simulink library "LumAerospaceBlockset_EquationsOfMotion"  (R2021a)
settings: Solver=ode45  StartTime=0.0  StopTime=10.0  RelTol=1e-3  EnableMultiTasking=on
values from neighbouring files (symbols this model uses):
  Xgeodetic0 = [lat0;lon0;h0]    [MAIN_RCAMDemo.m]
libraries: LumAerospaceBlockset_Utilities x3
settings Model: Creator=Christopher  LastModifiedBy=chris
settings SolverCC: AlgebraicLoopSolver=TrustRegion
settings DataIOCC: LimitDataPoints=on  SaveFormat=Array  ReturnWorkspaceOutputs=off
settings OptimizationCC: LifeSpan=inf
settings DebuggingCC: SolverPrmCheckMsg=warning  SFUnexpectedBacktrackingDiag=warning  SFNoUnconditionalDefaultTransitionDiag=warning  SFExecutionAtInitializationDiag=none  SFMachineParentedDataDiag=warning  ArithmeticOperatorsInVariantConditions=warning
settings HardwareCC: ProdBitPerPointer=32  ProdBitPerSizeT=32  ProdBitPerPtrDiffT=32  ProdLargestAtomicFloat=None  ProdIntDivRoundTo=Undefined  ProdEndianess=Unspecified  ProdWordSize=32  ProdHWDeviceType=32-bit Generic
settings ModelReferenceCC: PropagateSignalLabelsOutOfModel=off
settings SFSimCC: SimUseLocalCustomCode=off  CustomCodeUndefinedFunction=UseInterfaceOnly
settings RTWCC: RTWUseLocalCustomCode=off
settings CodeAppCC: StateflowObjectComments=on
settings GRTTargetCC: TargetLangStandard=C89/C90 (ANSI)
settings ConfigComp: CovMetricSettings=dw  CovSaveCumulativeToWorkspaceVar=on  CovSaveSingleToWorkspaceVar=on  CovExternalEMLEnable=off  CovSFcnEnable=off

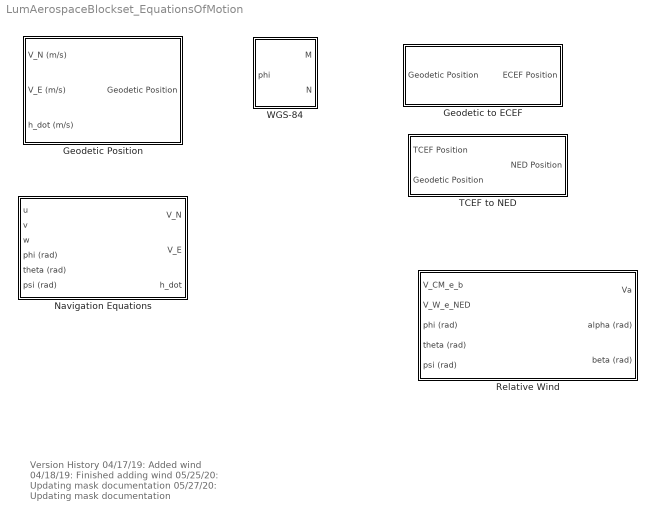
== system LumAerospaceBlockset_EquationsOfMotion ==
  note: Version History
      | 04/17/19: Added wind
      | 04/18/19: Finished adding wind
      | 05/25/20: Updating mask documentation
      | 05/27/20: Updating mask documentation
  Geodetic Position : Subsystem  mask{Xgeodetic0=Xgeodetic0}
      mask prompts: Xgeodetic0 "Initial Position (Geodetic)"
      mask help:
      | Obtains the position in Geodetic Coordinates from North-East-Down velocities.
      |
      | Longitude is bounded between [-pi,pi).  Latitutde is unbounded.  This creates problems near phi=+/-pi/2.  This block should not be used near these limits (ie north/south pole)
      |
      | Inputs are velocities in North-East-Down frame (except for h_dot = -V_down).    All inputs must be in units of meters/sec.
      |
      | Inputs:	V_N:	North velocity (m/s)
      | 	V_E:	East velocity (m/s)
      | 	h_dot:	Altitude_dot (m/s)
      |
      | Outputs:	3x1 vector of (phi;lambda;h).
      | 		phi = geodetic latitude (rad)
      | 		lambda = terrestrial longitude (rad)
      | 		h = geodetic altitude (m)
      |
      | For more information, see Stevens, B.L., Lewis, F.L., "Aircraft Control and Simulation 2nd Ed".  2003 John Wiley & Sons.  Pg. 37
      |
      | Christopher Lum
      | lum@uw.edu
  Geodetic to ECEF : Subsystem  Description=|
      | Version History  
      |                  
      | 05/??/05: Created
      mask help:
      | Convert from geodetic coordinates to Earth-Centered-Earth-Fixed (ECEF) frame.
      |
      | Inputs:		Geodetic Position:	3x1 vector of [phi;lambda;h].
      |
      | Outputs:	ECEF position:		3x1 vector of [x_ECEF;y_ECEF;z_ECEF].
      |
      | For more information, see Stevens, B.L., Lewis, F.L., "Aircraft Control and Simulation 2nd Ed".  2003 John Wiley & Sons.  Pg. 38
      |
      | Created by Christopher Lum
      | lum@u.washington.edu
  Navigation Equations : Subsystem  Description=|
      | Version History  
      |                  
      | 05/24/05: Created
      mask help:
      | Converts velocities in body frame to velocities in North-East-Down frame.  This computes the outputs using the following equations
      |
      | 	V_N = u*cos(theta)*cos(psi)+v*(-cos(phi)*sin(psi)+sin(phi)*sin(theta)*cos(psi))+w*(sin(phi)*sin(psi)+cos(phi)*sin(theta)*cos(psi))
      |
      | 	V_E = u*cos(theta)*sin(psi)+v*(cos(phi)*cos(psi)+sin(phi)*sin(theta)*sin(psi))+w*(-sin(phi)*cos(psi)+cos(phi)*sin(theta)*sin(psi))
      |
      | 	h_dot = u*sin(theta)-v*sin(phi)*cos(theta)-w*cos(phi)*cos(theta)
      |
      | Note that h_dot = -V_down
      |
      | Inputs:		u:	body velocity x
      | 		v:	body velocity y
      | 		w:	body velocity z
      | 		phi:	Euler angle bank (rad)
      | 		theta:	Euler angle pitch (rad)
      | 		psi:	Euler angle yaw (rad)
      |
      | Outputs:		V_N:	velocity north
      | 		V_E:	velocity east
      | 		h_dot:	altitude rate of change (positive h_dot implies climb)
      |
      | For more information, see Stevens, B.L., Lewis, F.L., "Aircraft Control and Simulation 2nd Ed". 2003 John Wiley & Sons. Pg.110
      |
      | Christopher Lum
      | lum@uw.edu
  Relative Wind : Subsystem
      mask help:
      | Computes the airspeed, angle of attack, and angle of sideslip experienced by an aircraft in a steady wind field.
      |
      | 	v_CM_e_b = [u;v;w]
      | 	V_W_e_NED   = [W_N; W_E; W_D]
      |
      | For example, if the wind is directly from the South (in other words it is blowing directly North) and 10 m/s, then V_W_e_n = [10; 0; 0].
      |
      | If there is no relative motion (V_CM_e_b = V_W_e_NED) then alpha and beta are set to 0 (as opposed to NaN).
      |
      | Inputs:	V_CM_e_b:	velocity vector of CM of aircraft w.r.t. earth/inertial frame expressed in the body (b) frame (3x1 vector)
      | 	V_W_e_NED:	velocity vector of the wind w.r.t. earth/inertial frame expressed in the north, east, down (NED) frame (3x1)
      | 	phi:	Euler angle bank (rad)
      | 	theta:	Euler angle pitch (rad)
      | 	psi:	Euler angle yaw (rad)
      |
      | Outputs:	Va:	airspeed experienced by the aircraft
      | 	alpha:	angle of attack experienced by aircraft (rad)
      | 	beta:	angle of sideslip experienced by aircraft (rad)
      |
      | Created by Christopher Lum
      | lum@uw.edu
      mask Display: image('WindIcon.png')
  TCEF to NED : Subsystem  Description=|
      | Version History  
      |                  
      | 05/??/05: Created
      mask help:
      | Convert from Target-Centered-Earth-Fixed (TCEF) frame to North-East-Down (NED) frame.  TCEF frame is same as ECEF frame except its origin is at target specified by phi, lambda, and h.
      |
      | Inputs:		TCEF Position:		3x1 vector of [x_TCEF;y_TCEF;z_TCEF].
      | 		Geodetic Position:	3x1 vector of [phi;lambda;h].
      |
      | Outputs:	NED position:		3x1 vector of [PN,PE,PD]
      |
      | For more information, see Stevens, B.L., Lewis, F.L., "Aircraft Control and Simulation 2nd Ed".  2003 John Wiley & Sons.  Pg. 37
      |
      | Created by Christopher Lum
      | lum@u.washington.edu
  WGS-84 : Subsystem  Description=|
      | Version History  
      |                  
      | 05/??/05: Created
      mask help:
      | Calculates the meridian raidus of curvature (M), and the prime vertical radius of curvature (N).
      |
      | Inputs:	phi:	Geodetic latitude (rad)
      |
      | Outputs:	M:	Meridian radius of curvature (m)
      | 	N:	Prime vertical radius of curvature (m)
      |
      | For more information, see Stevens, B.L., Lewis, F.L., "Aircraft Control and Simulation 2nd Ed".  2003 John Wiley & Sons.  Pg. 37
      |
      | Christopher Lum
      | lum@uw.edu

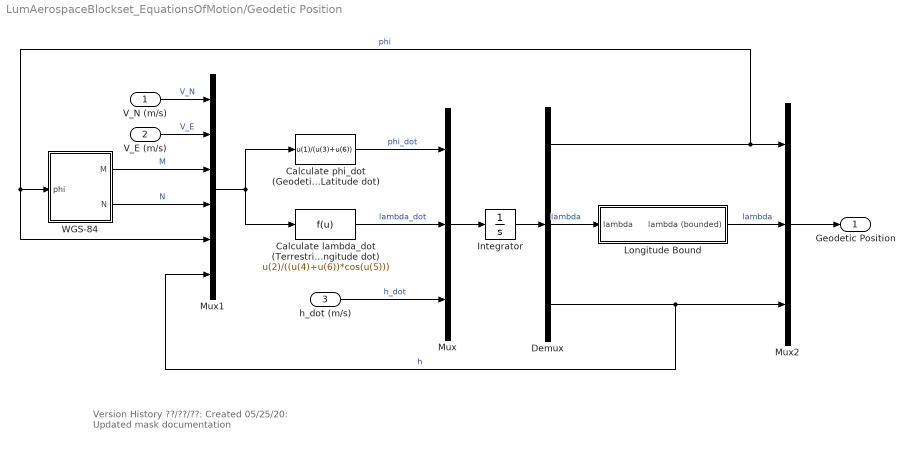
== system LumAerospaceBlockset_EquationsOfMotion/Geodetic Position ==
  note: Version History
      | ??/??/??: Created
      | 05/25/20: Updated mask documentation
  V_N (m/s) : Inport
  V_E (m/s) : Inport  Port=2
  h_dot (m/s) : Inport  Port=3
  Calculate lambda_dot (Terrestrial Longitude dot) : Fcn  Expr=u(2)/((u(4)+u(6))*cos(u(5)))
  Calculate phi_dot (Geodetic Latitude dot) : Fcn  Expr=u(1)/(u(3)+u(6))
  Demux : Demux  Outputs=3
  Integrator : Integrator  InitialCondition=Xgeodetic0
  Longitude Bound : Subsystem
      mask help:
      | Converts input longitude to it equivalent in the range [-pi,pi).
      |
      | Original Block concept from Aerosim Blockset by Unmanned Dynamics.  www.u-dynamics.com
  Mux : Mux  Inputs=3
  Mux1 : Mux  Inputs=6
  Mux2 : Mux  Inputs=3
  WGS-84 : Subsystem
  Geodetic Position : Outport  VectorParamsAs1DForOutWhenUnconnected=off
  wires:
  Longitude Bound/1(lambda (bounded)) -> Mux2/2  "lambda"
  Mux1/1 -> Calculate lambda_dot (Terrestrial Longitude dot)/1, Calculate phi_dot (Geodetic Latitude dot)/1
  Calculate phi_dot (Geodetic Latitude dot)/1 -> Mux/1  "phi_dot"
  Calculate lambda_dot (Terrestrial Longitude dot)/1 -> Mux/2  "lambda_dot"
  WGS-84/2(N) -> Mux1/4  "N"
  WGS-84/1("M ") -> Mux1/3  "M"
  h_dot (m/s)/1 -> Mux/3  "h_dot"
  V_E (m/s)/1 -> Mux1/2  "V_E"
  V_N (m/s)/1 -> Mux1/1  "V_N"
  Demux/3 -> Mux1/6, Mux2/3  "h"
  Demux/2 -> Longitude Bound/1(lambda)  "lambda"
  Demux/1 -> Mux1/5, WGS-84/1(phi), Mux2/1  "phi"
  Integrator/1 -> Demux/1
  Mux/1 -> Integrator/1
  Mux2/1 -> Geodetic Position/1

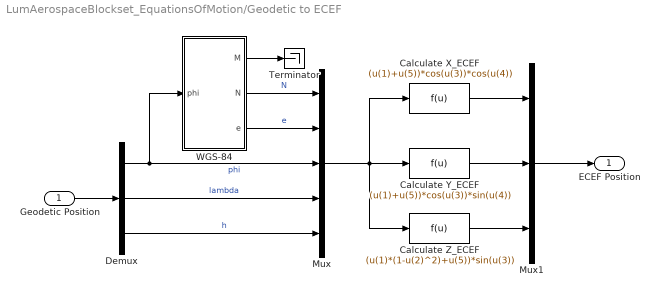
== system LumAerospaceBlockset_EquationsOfMotion/Geodetic to ECEF ==
  Geodetic Position : Inport
  Calculate X_ECEF : Fcn  Expr=(u(1)+u(5))*cos(u(3))*cos(u(4))
  Calculate Y_ECEF : Fcn  Expr=(u(1)+u(5))*cos(u(3))*sin(u(4))
  Calculate Z_ECEF : Fcn  Expr=(u(1)*(1-u(2)^2)+u(5))*sin(u(3))
  Demux : Demux  Outputs=3
  Mux : Mux  Inputs=5
  Mux1 : Mux  Inputs=3
  Terminator : Terminator
  WGS-84 : Subsystem
  ECEF Position : Outport  VectorParamsAs1DForOutWhenUnconnected=off
  wires:
  Geodetic Position/1 -> Demux/1
  Mux/1 -> Calculate Y_ECEF/1, Calculate X_ECEF/1, Calculate Z_ECEF/1
  Calculate X_ECEF/1 -> Mux1/1
  Calculate Y_ECEF/1 -> Mux1/2
  Calculate Z_ECEF/1 -> Mux1/3
  Mux1/1 -> ECEF Position/1
  Demux/2 -> Mux/4  "lambda"
  Demux/3 -> Mux/5  "h"
  WGS-84/2(N) -> Mux/1  "N"
  WGS-84/3(e) -> Mux/2  "e"
  Demux/1 -> Mux/3, WGS-84/1(phi)  "phi"
  WGS-84/1("M ") -> Terminator/1

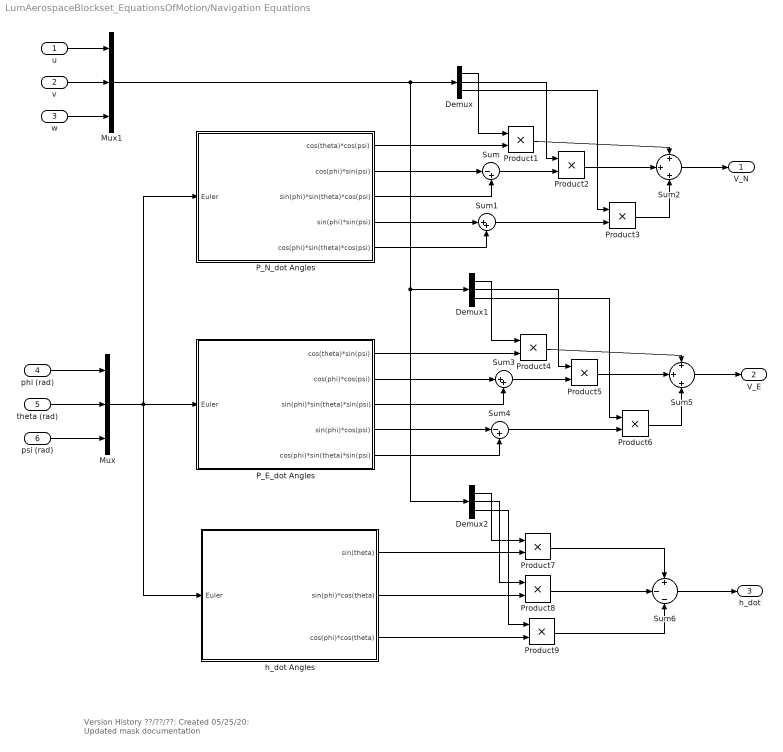
== system LumAerospaceBlockset_EquationsOfMotion/Navigation Equations ==
  note: Version History
      | ??/??/??: Created
      | 05/25/20: Updated mask documentation
  u : Inport
  v : Inport  Port=2
  w : Inport  Port=3
  phi (rad) : Inport  Port=4
  theta (rad) : Inport  Port=5
  psi (rad) : Inport  Port=6
  Demux : Demux  Outputs=3
  Demux1 : Demux  Outputs=3
  Demux2 : Demux  Outputs=3
  Mux : Mux  Inputs=3
  Mux1 : Mux  Inputs=3
  P_E_dot Angles : Subsystem
  P_N_dot Angles : Subsystem
  Product{1..9} (9 alike) : Product  RndMeth=Zero
  Sum : Sum  Inputs=|-+
  Sum1 : Sum  Inputs=|++
  Sum2 : Sum  Inputs=+|+|+
  Sum3 : Sum  Inputs=|++
  Sum4 : Sum  Inputs=|-+
  Sum5 : Sum  Inputs=+|+|+
  Sum6 : Sum  Inputs=+|-|-
  h_dot Angles : Subsystem
  V_N : Outport  VectorParamsAs1DForOutWhenUnconnected=off
  V_E : Outport  Port=2  VectorParamsAs1DForOutWhenUnconnected=off
  h_dot : Outport  Port=3  VectorParamsAs1DForOutWhenUnconnected=off
  wires:
  Sum6/1 -> h_dot/1
  Product9/1 -> Sum6/3
  Product8/1 -> Sum6/2
  Product7/1 -> Sum6/1
  h_dot Angles/3(cos(phi)*cos(theta)) -> Product9/2
  Demux2/3 -> Product9/1
  h_dot Angles/2(sin(phi)*cos(theta)) -> Product8/2
  Demux2/2 -> Product8/1
  h_dot Angles/1(sin(theta)) -> Product7/2
  Demux2/1 -> Product7/1
  P_E_dot Angles/5(cos(phi)*sin(theta)*sin(psi)) -> Sum4/2
  P_E_dot Angles/4(sin(phi)*cos(psi)) -> Sum4/1
  P_E_dot Angles/3(sin(phi)*sin(theta)*sin(psi)) -> Sum3/2
  P_E_dot Angles/2(cos(phi)*cos(psi)) -> Sum3/1
  P_E_dot Angles/1(cos(theta)*sin(psi)) -> Product4/2
  Demux1/3 -> Product6/1
  Demux1/2 -> Product5/1
  Demux1/1 -> Product4/1
  Sum5/1 -> V_E/1
  Product6/1 -> Sum5/3
  Product5/1 -> Sum5/2
  Product4/1 -> Sum5/1
  Sum4/1 -> Product6/2
  Sum3/1 -> Product5/2
  Demux/3 -> Product3/1
  Demux/2 -> Product2/1
  Demux/1 -> Product1/1
  Mux1/1 -> Demux2/1, Demux1/1, Demux/1
  w/1 -> Mux1/3
  v/1 -> Mux1/2
  u/1 -> Mux1/1
  Sum2/1 -> V_N/1
  Product3/1 -> Sum2/3
  Product2/1 -> Sum2/2
  Product1/1 -> Sum2/1
  Sum1/1 -> Product3/2
  P_N_dot Angles/5(cos(phi)*sin(theta)*cos(psi)) -> Sum1/2
  P_N_dot Angles/4(sin(phi)*sin(psi)) -> Sum1/1
  Sum/1 -> Product2/2
  P_N_dot Angles/3(sin(phi)*sin(theta)*cos(psi)) -> Sum/2
  P_N_dot Angles/2("cos(phi)*sin(psi) ") -> Sum/1
  P_N_dot Angles/1(cos(theta)*cos(psi)) -> Product1/2
  Mux/1 -> h_dot Angles/1(Euler), P_E_dot Angles/1(Euler), P_N_dot Angles/1(Euler)
  psi (rad)/1 -> Mux/3
  theta (rad)/1 -> Mux/2
  phi (rad)/1 -> Mux/1

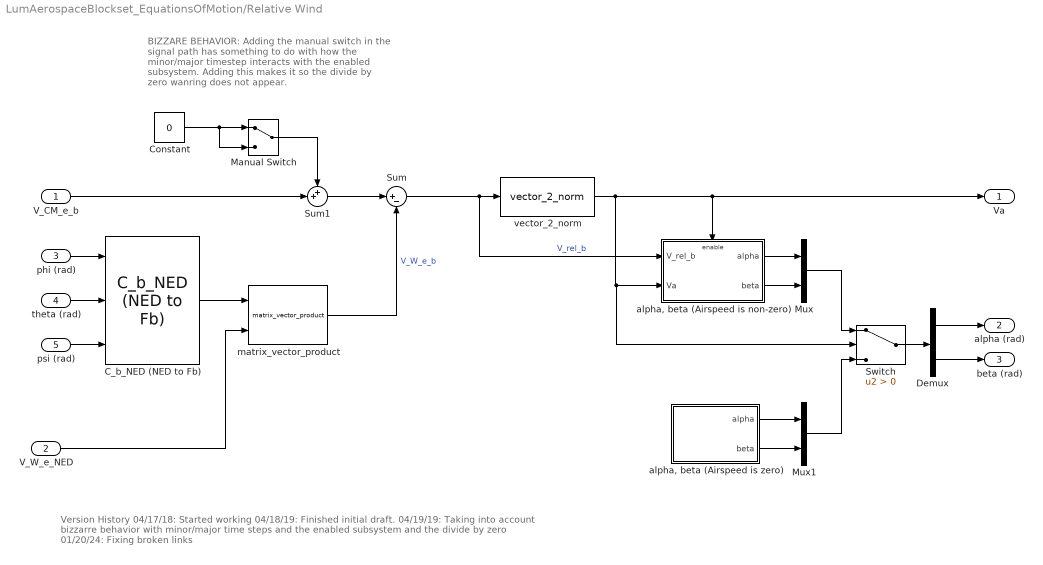
== system LumAerospaceBlockset_EquationsOfMotion/Relative Wind ==
  note: BIZZARE BEHAVIOR: Adding the manual switch in the signal path has something to do with how the minor/major timestep interacts with the enabled subsystem. Adding this makes it so the divide by zero wanring does not appear.
  note: Version History
      | 04/17/18: Started working
      | 04/18/19: Finished initial draft.
      | 04/19/19: Taking into account bizzarre behavior with minor/major time steps and the enabled subsystem and the divide by zero
      | 01/20/24: Fixing broken links
  V_CM_e_b : Inport
  V_W_e_NED : Inport  Port=2
  phi (rad) : Inport  Port=3
  theta (rad) : Inport  Port=4
  psi (rad) : Inport  Port=5
  C_b_NED (NED to Fb) : LumAerospaceBlockset_Utilities/C_b_NED (NED to Fb)
  Constant : Constant  Value=0
  Demux : Demux  Outputs=2
  Manual Switch : ManualSwitch
  Mux : Mux  Inputs=2
  Mux1 : Mux  Inputs=2
  Sum : Sum  Inputs=|+-
  Sum1 : Sum  Inputs=++|
  Switch : Switch  Criteria=u2 > Threshold
  "alpha, beta (Airspeed is non-zero)" : Subsystem
  "alpha, beta (Airspeed is zero)" : Subsystem
  matrix_vector_product : LumAerospaceBlockset_Utilities/matrix_vector_product
  vector_2_norm : LumAerospaceBlockset_Utilities/vector_2_norm
  Va : Outport  VectorParamsAs1DForOutWhenUnconnected=off
  alpha (rad) : Outport  Port=2  VectorParamsAs1DForOutWhenUnconnected=off
  beta (rad) : Outport  Port=3  VectorParamsAs1DForOutWhenUnconnected=off
  wires:
  V_W_e_NED/1 -> matrix_vector_product/2
  V_CM_e_b/1 -> Sum1/2
  Sum/1 -> "alpha, beta (Airspeed is non-zero)"/1(V_rel_b), vector_2_norm/1  "V_rel_b"
  psi (rad)/1 -> C_b_NED (NED to Fb)/3
  phi (rad)/1 -> C_b_NED (NED to Fb)/1
  theta (rad)/1 -> C_b_NED (NED to Fb)/2
  C_b_NED (NED to Fb)/1 -> matrix_vector_product/1
  matrix_vector_product/1 -> Sum/2  "V_W_e_b"
  "alpha, beta (Airspeed is non-zero)"/1(alpha) -> Mux/1
  "alpha, beta (Airspeed is non-zero)"/2(beta) -> Mux/2
  "alpha, beta (Airspeed is zero)"/1(alpha) -> Mux1/1
  "alpha, beta (Airspeed is zero)"/2(beta) -> Mux1/2
  vector_2_norm/1 -> Switch/2, "alpha, beta (Airspeed is non-zero)"/2(Va), Va/1, "alpha, beta (Airspeed is non-zero)"/Enable
  Mux/1 -> Switch/1
  Mux1/1 -> Switch/3
  Switch/1 -> Demux/1
  Demux/1 -> alpha (rad)/1
  Demux/2 -> beta (rad)/1
  Manual Switch/1 -> Sum1/1
  Constant/1 -> Manual Switch/2, Manual Switch/1
  Sum1/1 -> Sum/1

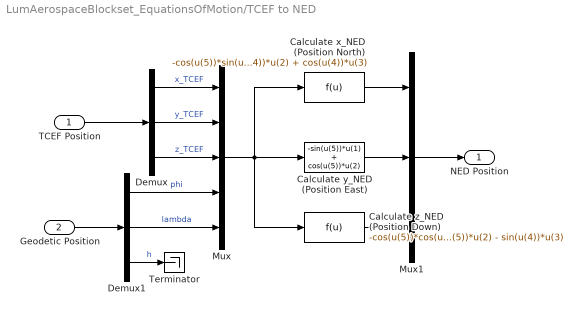
== system LumAerospaceBlockset_EquationsOfMotion/TCEF to NED ==
  TCEF Position : Inport
  Geodetic Position : Inport  Port=2
  Calculate x_NED (Position North) : Fcn  Expr=-cos(u(5))*sin(u(4))*u(1) - sin(u(5))*sin(u(4))*u(2) + cos(u(4))*u(3)
  Calculate y_NED (Position East) : Fcn  Expr=-sin(u(5))*u(1) + cos(u(5))*u(2)
  Calculate z_NED (Position Down) : Fcn  Expr=-cos(u(5))*cos(u(4))*u(1) - cos(u(4))*sin(u(5))*u(2) - sin(u(4))*u(3)
  Demux : Demux  Outputs=3
  Demux1 : Demux  Outputs=3
  Mux : Mux  Inputs=5
  Mux1 : Mux  Inputs=3
  Terminator : Terminator
  NED Position : Outport  VectorParamsAs1DForOutWhenUnconnected=off
  wires:
  TCEF Position/1 -> Demux/1
  Geodetic Position/1 -> Demux1/1
  Demux/1 -> Mux/1  "x_TCEF"
  Demux/2 -> Mux/2  "y_TCEF"
  Demux/3 -> Mux/3  "z_TCEF"
  Demux1/1 -> Mux/4  "phi"
  Demux1/2 -> Mux/5  "lambda"
  Demux1/3 -> Terminator/1  "h"
  Calculate x_NED (Position North)/1 -> Mux1/1
  Calculate y_NED (Position East)/1 -> Mux1/2
  Calculate z_NED (Position Down)/1 -> Mux1/3
  Mux1/1 -> NED Position/1
  Mux/1 -> Calculate y_NED (Position East)/1, Calculate x_NED (Position North)/1, Calculate z_NED (Position Down)/1

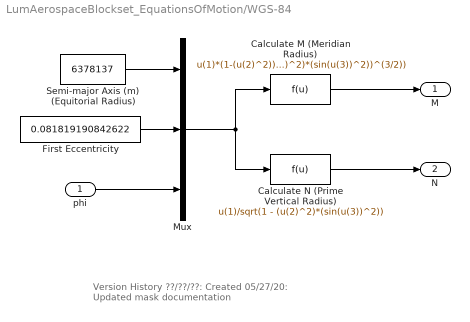
== system LumAerospaceBlockset_EquationsOfMotion/WGS-84 ==
  note: Version History
      | ??/??/??: Created
      | 05/27/20: Updated mask documentation
  phi : Inport
  Calculate M (Meridian Radius) : Fcn  Expr=u(1)*(1-(u(2)^2))/((1-(u(2)^2)*(sin(u(3))^2))^(3/2))
  Calculate N (Prime Vertical Radius) : Fcn  Expr=u(1)/sqrt(1 - (u(2)^2)*(sin(u(3))^2))
  First Eccentricity : Constant  Value=0.081819190842622
  Mux : Mux  Inputs=3
  "Semi-major Axis (m) (Equitorial Radius) " : Constant  Value=6378137
  "M " : Outport  VectorParamsAs1DForOutWhenUnconnected=off
  N : Outport  Port=2  VectorParamsAs1DForOutWhenUnconnected=off
  wires:
  "Semi-major Axis (m) (Equitorial Radius) "/1 -> Mux/1
  First Eccentricity/1 -> Mux/2
  Calculate M (Meridian Radius)/1 -> "M "/1
  phi/1 -> Mux/3
  Calculate N (Prime Vertical Radius)/1 -> N/1
  Mux/1 -> Calculate N (Prime Vertical Radius)/1, Calculate M (Meridian Radius)/1

== system LumAerospaceBlockset_EquationsOfMotion/Geodetic Position/Longitude Bound ==
  lambda : Inport
  2pi : Constant  Value=2*pi
  Math Function : Math  Operator=mod  SignedPower=on  SaturateOnIntegerOverflow=on
  Sum1 : Sum  Inputs=|+-  InputSameDT=on  SaturateOnIntegerOverflow=on  OutDataTypeStr=Inherit: Same as first input
  Sum2 : Sum  Inputs=|++  InputSameDT=on  SaturateOnIntegerOverflow=on  OutDataTypeStr=Inherit: Same as first input
  pi : Constant  Value=pi
  lambda (bounded) : Outport  VectorParamsAs1DForOutWhenUnconnected=off
  wires:
  Sum1/1 -> lambda (bounded)/1
  lambda/1 -> Sum2/1
  pi/1 -> Sum1/2, Sum2/2
  Sum2/1 -> Math Function/1
  2pi/1 -> Math Function/2
  Math Function/1 -> Sum1/1

== system LumAerospaceBlockset_EquationsOfMotion/Geodetic Position/WGS-84 ==
  phi : Inport
  Calculate M (Meridian Radius) : Fcn  Expr=u(1)*(1-(u(2)^2))/((1-(u(2)^2)*(sin(u(3))^2))^(3/2))
  Calculate N (Prime Vertical Radius) : Fcn  Expr=u(1)/sqrt(1 - (u(2)^2)*(sin(u(3))^2))
  First Eccentricity : Constant  Value=0.081819190842622
  Mux : Mux  Inputs=3
  "Semi-major Axis (m) (Equitorial Radius) " : Constant  Value=6378137
  "M " : Outport  VectorParamsAs1DForOutWhenUnconnected=off
  N : Outport  Port=2  VectorParamsAs1DForOutWhenUnconnected=off
  wires:
  Mux/1 -> Calculate M (Meridian Radius)/1, Calculate N (Prime Vertical Radius)/1
  Calculate N (Prime Vertical Radius)/1 -> N/1
  phi/1 -> Mux/3
  Calculate M (Meridian Radius)/1 -> "M "/1
  First Eccentricity/1 -> Mux/2
  "Semi-major Axis (m) (Equitorial Radius) "/1 -> Mux/1

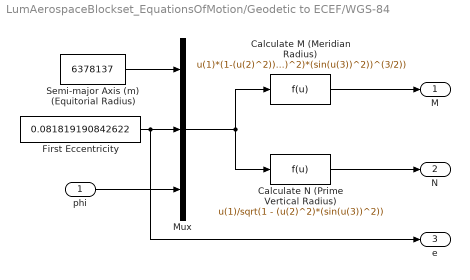
== system LumAerospaceBlockset_EquationsOfMotion/Geodetic to ECEF/WGS-84 ==
  phi : Inport
  Calculate M (Meridian Radius) : Fcn  Expr=u(1)*(1-(u(2)^2))/((1-(u(2)^2)*(sin(u(3))^2))^(3/2))
  Calculate N (Prime Vertical Radius) : Fcn  Expr=u(1)/sqrt(1 - (u(2)^2)*(sin(u(3))^2))
  First Eccentricity : Constant  Value=0.081819190842622
  Mux : Mux  Inputs=3
  "Semi-major Axis (m) (Equitorial Radius) " : Constant  Value=6378137
  "M " : Outport  VectorParamsAs1DForOutWhenUnconnected=off
  N : Outport  Port=2  VectorParamsAs1DForOutWhenUnconnected=off
  e : Outport  Port=3  VectorParamsAs1DForOutWhenUnconnected=off
  wires:
  Mux/1 -> Calculate M (Meridian Radius)/1, Calculate N (Prime Vertical Radius)/1
  Calculate N (Prime Vertical Radius)/1 -> N/1
  phi/1 -> Mux/3
  Calculate M (Meridian Radius)/1 -> "M "/1
  First Eccentricity/1 -> Mux/2, e/1
  "Semi-major Axis (m) (Equitorial Radius) "/1 -> Mux/1

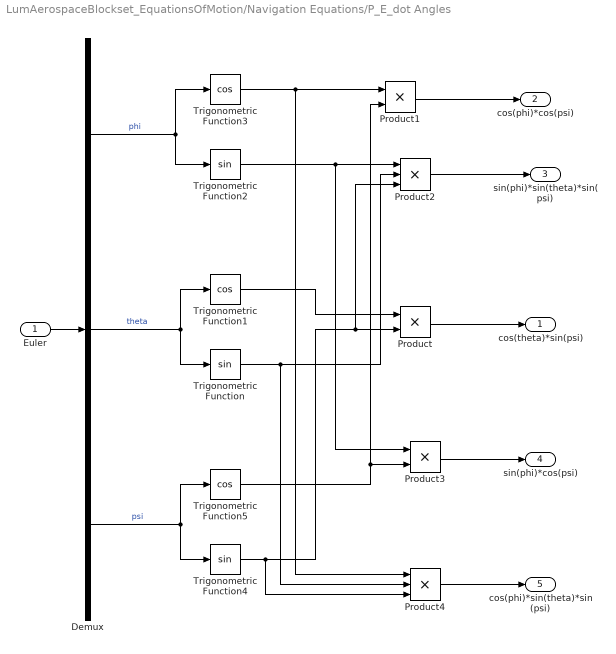
== system LumAerospaceBlockset_EquationsOfMotion/Navigation Equations/P_E_dot Angles ==
  Euler : Inport
  Demux : Demux  Outputs=3
  Product : Product  RndMeth=Zero
  Product1 : Product  RndMeth=Zero
  Product2 : Product  Inputs=3  RndMeth=Zero
  Product3 : Product  RndMeth=Zero
  Product4 : Product  Inputs=3  RndMeth=Zero
  Trigonometric Function : Trigonometry
  Trigonometric Function1 : Trigonometry  Operator=cos
  Trigonometric Function2 : Trigonometry
  Trigonometric Function3 : Trigonometry  Operator=cos
  Trigonometric Function4 : Trigonometry
  Trigonometric Function5 : Trigonometry  Operator=cos
  cos(theta)*sin(psi) : Outport  VectorParamsAs1DForOutWhenUnconnected=off
  cos(phi)*cos(psi) : Outport  Port=2  VectorParamsAs1DForOutWhenUnconnected=off
  sin(phi)*sin(theta)*sin(psi) : Outport  Port=3  VectorParamsAs1DForOutWhenUnconnected=off
  sin(phi)*cos(psi) : Outport  Port=4  VectorParamsAs1DForOutWhenUnconnected=off
  cos(phi)*sin(theta)*sin(psi) : Outport  Port=5  VectorParamsAs1DForOutWhenUnconnected=off
  wires:
  Trigonometric Function/1 -> Product4/2, Product2/2
  Trigonometric Function2/1 -> Product3/1, Product2/1
  Trigonometric Function5/1 -> Product3/2, Product1/2
  Trigonometric Function3/1 -> Product4/1, Product1/1
  Trigonometric Function4/1 -> Product4/3, Product2/3, Product/2
  Trigonometric Function1/1 -> Product/1
  Demux/1 -> Trigonometric Function2/1, Trigonometric Function3/1  "phi"
  Demux/2 -> Trigonometric Function/1, Trigonometric Function1/1  "theta"
  Demux/3 -> Trigonometric Function4/1, Trigonometric Function5/1  "psi"
  Product/1 -> cos(theta)*sin(psi)/1
  Product1/1 -> cos(phi)*cos(psi)/1
  Product2/1 -> sin(phi)*sin(theta)*sin(psi)/1
  Product3/1 -> sin(phi)*cos(psi)/1
  Product4/1 -> cos(phi)*sin(theta)*sin(psi)/1
  Euler/1 -> Demux/1

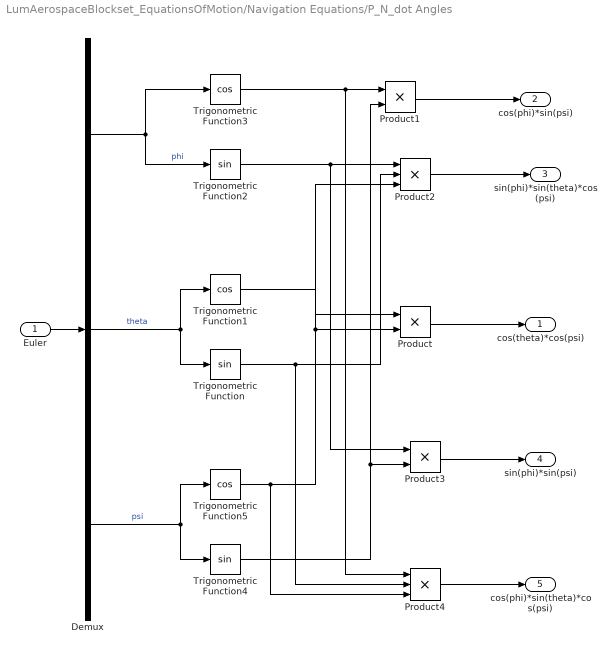
== system LumAerospaceBlockset_EquationsOfMotion/Navigation Equations/P_N_dot Angles ==
  Euler : Inport
  Demux : Demux  Outputs=3
  Product : Product  RndMeth=Zero
  Product1 : Product  RndMeth=Zero
  Product2 : Product  Inputs=3  RndMeth=Zero
  Product3 : Product  RndMeth=Zero
  Product4 : Product  Inputs=3  RndMeth=Zero
  Trigonometric Function : Trigonometry
  Trigonometric Function1 : Trigonometry  Operator=cos
  Trigonometric Function2 : Trigonometry
  Trigonometric Function3 : Trigonometry  Operator=cos
  Trigonometric Function4 : Trigonometry
  Trigonometric Function5 : Trigonometry  Operator=cos
  cos(theta)*cos(psi) : Outport  VectorParamsAs1DForOutWhenUnconnected=off
  "cos(phi)*sin(psi) " : Outport  Port=2  VectorParamsAs1DForOutWhenUnconnected=off
  sin(phi)*sin(theta)*cos(psi) : Outport  Port=3  VectorParamsAs1DForOutWhenUnconnected=off
  sin(phi)*sin(psi) : Outport  Port=4  VectorParamsAs1DForOutWhenUnconnected=off
  cos(phi)*sin(theta)*cos(psi) : Outport  Port=5  VectorParamsAs1DForOutWhenUnconnected=off
  wires:
  Euler/1 -> Demux/1
  Demux/1 -> Trigonometric Function2/1, Trigonometric Function3/1  "phi"
  Product4/1 -> cos(phi)*sin(theta)*cos(psi)/1
  Product3/1 -> sin(phi)*sin(psi)/1
  Trigonometric Function/1 -> Product4/2, Product2/2
  Product2/1 -> sin(phi)*sin(theta)*cos(psi)/1
  Trigonometric Function2/1 -> Product3/1, Product2/1
  Product1/1 -> "cos(phi)*sin(psi) "/1
  Trigonometric Function4/1 -> Product3/2, Product1/2
  Trigonometric Function3/1 -> Product4/1, Product1/1
  Product/1 -> cos(theta)*cos(psi)/1
  Trigonometric Function5/1 -> Product4/3, Product2/3, Product/2
  Trigonometric Function1/1 -> Product/1
  Demux/3 -> Trigonometric Function5/1, Trigonometric Function4/1  "psi"
  Demux/2 -> Trigonometric Function1/1, Trigonometric Function/1  "theta"

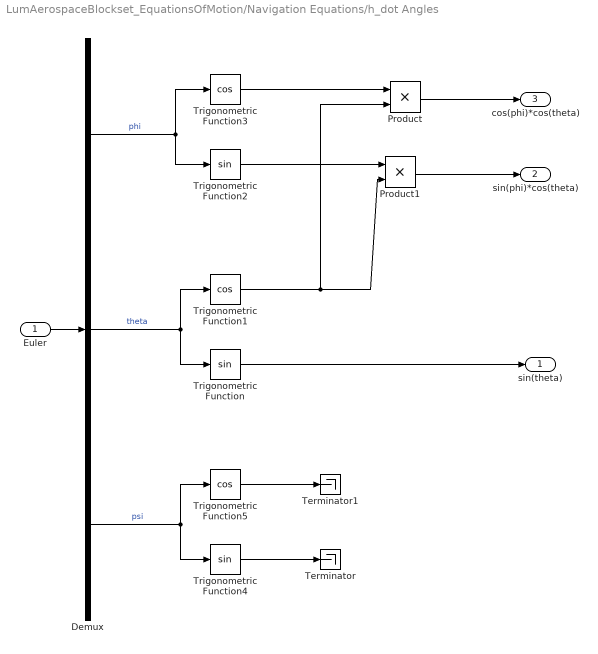
== system LumAerospaceBlockset_EquationsOfMotion/Navigation Equations/h_dot Angles ==
  Euler : Inport
  Demux : Demux  Outputs=3
  Product : Product  RndMeth=Zero
  Product1 : Product  RndMeth=Zero
  Terminator : Terminator
  Terminator1 : Terminator
  Trigonometric Function : Trigonometry
  Trigonometric Function1 : Trigonometry  Operator=cos
  Trigonometric Function2 : Trigonometry
  Trigonometric Function3 : Trigonometry  Operator=cos
  Trigonometric Function4 : Trigonometry
  Trigonometric Function5 : Trigonometry  Operator=cos
  sin(theta) : Outport  VectorParamsAs1DForOutWhenUnconnected=off
  sin(phi)*cos(theta) : Outport  Port=2  VectorParamsAs1DForOutWhenUnconnected=off
  cos(phi)*cos(theta) : Outport  Port=3  VectorParamsAs1DForOutWhenUnconnected=off
  wires:
  Trigonometric Function5/1 -> Terminator1/1
  Product/1 -> cos(phi)*cos(theta)/1
  Trigonometric Function3/1 -> Product/1
  Trigonometric Function1/1 -> Product/2, Product1/2
  Trigonometric Function2/1 -> Product1/1
  Euler/1 -> Demux/1
  Product1/1 -> sin(phi)*cos(theta)/1
  Demux/3 -> Trigonometric Function5/1, Trigonometric Function4/1  "psi"
  Demux/2 -> Trigonometric Function1/1, Trigonometric Function/1  "theta"
  Demux/1 -> Trigonometric Function3/1, Trigonometric Function2/1  "phi"
  Trigonometric Function4/1 -> Terminator/1
  Trigonometric Function/1 -> sin(theta)/1

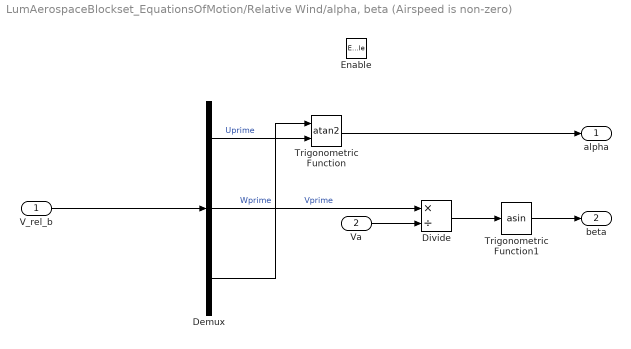
== system LumAerospaceBlockset_EquationsOfMotion/Relative Wind/alpha, beta (Airspeed is non-zero) ==
  V_rel_b : Inport
  Va : Inport  Port=2
  Enable : EnablePort
  Demux : Demux  Outputs=3
  Divide : Product  Inputs=*/
  Trigonometric Function : Trigonometry  Operator=atan2
  Trigonometric Function1 : Trigonometry  Operator=asin
  alpha : Outport  VectorParamsAs1DForOutWhenUnconnected=off
  beta : Outport  Port=2  VectorParamsAs1DForOutWhenUnconnected=off
  wires:
  Demux/2 -> Divide/1  "Vprime"
  Demux/1 -> Trigonometric Function/2  "Uprime"
  Demux/3 -> Trigonometric Function/1  "Wprime"
  Divide/1 -> Trigonometric Function1/1
  Va/1 -> Divide/2
  Trigonometric Function/1 -> alpha/1
  V_rel_b/1 -> Demux/1
  Trigonometric Function1/1 -> beta/1

== system LumAerospaceBlockset_EquationsOfMotion/Relative Wind/alpha, beta (Airspeed is zero) ==
  Constant : Constant  Value=0
  alpha : Outport  VectorParamsAs1DForOutWhenUnconnected=off
  beta : Outport  Port=2  VectorParamsAs1DForOutWhenUnconnected=off
  wires:
  Constant/1 -> alpha/1, beta/1
